simulink model "Kalman_Filter_ETR07"  (R2017b)
settings: Solver=VariableStepAuto  StartTime=0.0  StopTime=10.0  RelTol=1e-3
settings Model: Creator=cspt  LastModifiedBy=cspt

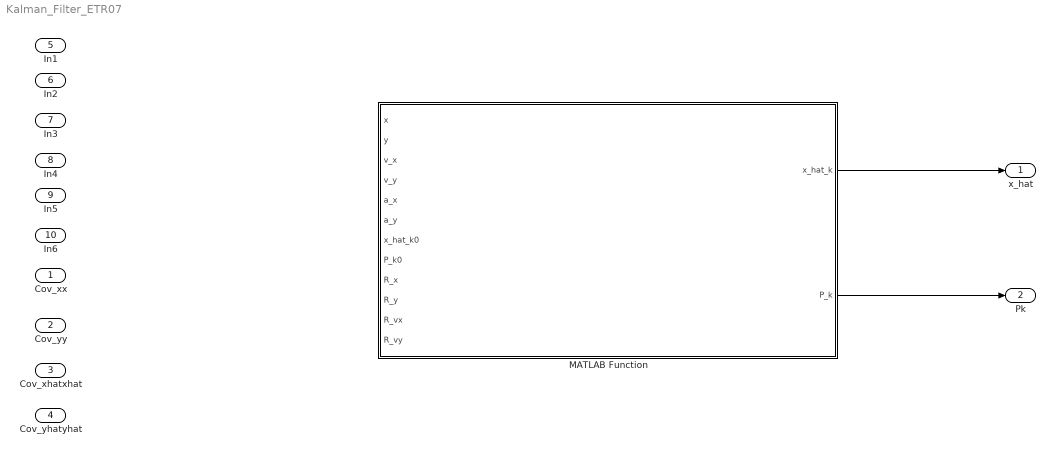
== system Kalman_Filter_ETR07 ==
  Cov_xx : Inport
  "Cov_yy " : Inport  Port=2
  Cov_xhatxhat : Inport  Port=3
  Cov_yhatyhat : Inport  Port=4
  In1 : Inport  Port=5
  In2 : Inport  Port=6
  In3 : Inport  Port=7
  In4 : Inport  Port=8
  In5 : Inport  Port=9
  In6 : Inport  Port=10
  MATLAB Function : MATLAB Function  TreatAsAtomicUnit=on
  x_hat : Outport
  Pk : Outport  Port=2
  wires:
  MATLAB Function/1(x_hat_k) -> x_hat/1
  MATLAB Function/2(P_k) -> Pk/1

== matlab function Kalman_Filter_ETR07/MATLAB Function ==
  data: x input; x_hat_k output; y input; v_x input; v_y input; a_x input; a_y input; x_hat_k0 input; P_k output; P_k0 input; R_x input; R_y input; R_vx input; R_vy input
function [x_hat_k,P_k] = kf(x, y, v_x, v_y, a_x, a_y, x_hat_k0, P_k0, R_x, R_y, R_vx, R_vy)

    %A matrix
    A = [1 0 -Ts 0; 0 1 0 -Ts; 0 0 1 0; 0 0 0 1];

    %B matrix
    B = [1/2*(-Ts^2); -Ts^2];

    %C matrix
    C = [1 0 0 0; 0 1 0 0; 0 0 1 0; 0 0 0 1];

    %Identity matrix
    I = [1 0 0 0; 0 1 0 0; 0 0 1 0; 0 0 0 1];

    %Process noise covariance R
    R = [R_x 0 0 0; 0 R_y 0 0; 0 0 R_vx 0; 0 0 0 R_vy];

    %Process noise covariance Q
    Q = [0.02 0 0 0; 0 0.02 0 0; 0 0 0.01 0; 0 0 0 0.04];

    %Uk matrix
    u_k = [a_x; a_y];

    %y_k matrix
    y_k = [x; y; v_x; v_y];

    x_hat_ = A*x_hat_k0 + B*u_k;

    P_k_ = A*P_k0*A' + Q;

    %Kalman constant calculation
    S = C*P_k_*C' + R;
    K_k = (P_k_*C')/S;

    %x_hat and Covariance calculation
    x_hat_k = x_hat_ + K_k*(y_k - C*x_hat_);
    P_k = (I - K_k*C)*P_k_;
end
